simulink model "Linear_Model_Validation"  (R2019b)
settings: Solver=FixedStepAuto  StartTime=0.0  StopTime=10.0  MaxStep=0.025  RelTol=1e-3
values from neighbouring files (symbols this model uses):
  A = [-(Cf+Cr)/(m*Vx), -1-(lf*Cf-lr*Cr)/(m*Vx^2) ... (first row only)    [Mz_input_Model_Validation.m]    (also in TestData_DLC_u85_v60.mat = [6.9152159257  -1.26405171152; -375.707204017  87.7555625953)
  B = [Cf/(m*Vx) 0;(lf*Cf)/Iz 1/Iz]    [Mz_input_Model_Validation.m]    (also in TestData_DLC_u85_v60.mat = [-2.30062890982  0; -275.450986629  0.00311526479751])
settings Model: Creator=Shouvik Chakraborty  LastModifiedBy=Shouvik Chakraborty
settings SFSimCC: CustomCodeUndefinedFunction=UseInterfaceOnly

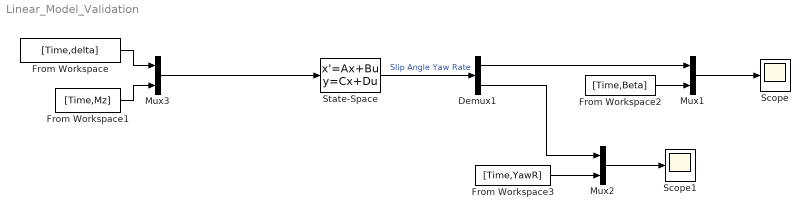
== system Linear_Model_Validation ==
  Demux1 : Demux  Outputs=2
  From Workspace : FromWorkspace  VariableName=[Time,delta]  SampleTime=0
  From Workspace1 : FromWorkspace  VariableName=[Time,Mz]  SampleTime=0
  From Workspace2 : FromWorkspace  VariableName=[Time,Beta]  SampleTime=0
  From Workspace3 : FromWorkspace  VariableName=[Time,YawR]  SampleTime=0
  Mux1 : Mux  Inputs=2
  Mux2 : Mux  Inputs=2
  Mux3 : Mux  Inputs=2
  Scope : Scope
  Scope1 : Scope
  State-Space : StateSpace  A=A  B=B  C=eye(2)  D=[0 0;0 0]  InitialCondition=0
  wires:
  State-Space/1 -> Demux1/1  "Slip Angle Yaw Rate"
  Mux3/1 -> State-Space/1
  Demux1/1 -> Mux1/1
  Demux1/2 -> Mux2/1
  Mux1/1 -> Scope/1
  Mux2/1 -> Scope1/1
  From Workspace/1 -> Mux3/1
  From Workspace1/1 -> Mux3/2
  From Workspace2/1 -> Mux1/2
  From Workspace3/1 -> Mux2/2
